simulink model "exp4"  (R2019a)
settings: Solver=ode45  StartTime=0.0  StopTime=10.0  RelTol=1e-3
values from neighbouring files (symbols this model uses):
  Kd = 0.1    [launcher.m]
  Kdp = 0.1    [launcher.m]
  Ki = 0.2    [launcher.m]
  Kip = 0.2    [launcher.m]
  Kp = 5.0    (= 5)    [launcher.m]
  Kpp = 5.0    (= 5)    [launcher.m]
settings Model: Creator=hlf  LastModifiedBy=Aaron
settings DataIOCC: SaveFormat=StructureWithTime
settings OptimizationCC: LifeSpan=inf
settings DebuggingCC: SFExecutionAtInitializationDiag=none  ArithmeticOperatorsInVariantConditions=warning
settings HardwareCC: ProdBitPerSizeT=32  ProdBitPerPtrDiffT=32  ProdWordSize=32  ProdHWDeviceType=Specified
settings CodeAppCC: StateflowObjectComments=on

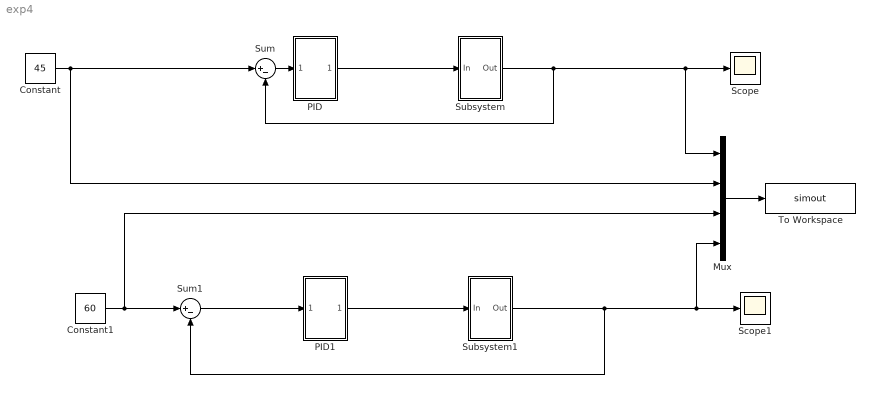
== system exp4 ==
  Constant : Constant  Value=45
  Constant1 : Constant  Value=60
  Mux : Mux
  PID : Subsystem
  PID1 : Subsystem
  Scope : Scope
  Scope1 : Scope
  Subsystem : Subsystem  mask{Ka=0.004, Kf=0.25, Vm=10e-6, Dm=1.75e-5, Kq=0.043, betae=7e8, Kce=3e-13, Jt=0.0167}
  Subsystem1 : Subsystem  mask{Ka=0.004, Kf=0.25, Vm=10e-6, Dm=1.75e-5, Kq=0.043, betae=7e8, Kce=3e-13, Jt=0.0167}
  Sum : Sum  Inputs=|+-
  Sum1 : Sum  Inputs=|+-
  To Workspace : ToWorkspace  VariableName=simout  SaveFormat=Timeseries  SampleTime=-1
  wires:
  Sum/1 -> PID/1(In1)
  PID/1(Out1) -> Subsystem/1(In)
  Subsystem1/1(Out) -> Sum1/2, Mux/4, Scope1/1
  PID1/1(Out1) -> Subsystem1/1(In)
  Sum1/1 -> PID1/1(In1)
  Constant1/1 -> Mux/3, Sum1/1
  Subsystem/1(Out) -> Mux/1, Scope/1, Sum/2
  Mux/1 -> To Workspace/1
  Constant/1 -> Sum/1, Mux/2

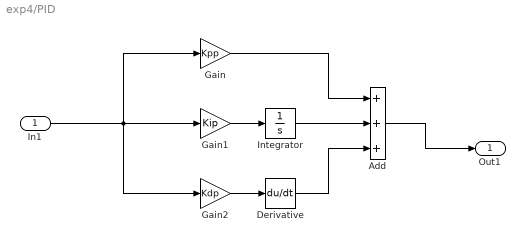
== system exp4/PID ==
  In1 : Inport
  Add : Sum  Inputs=+++
  Derivative : Derivative
  Gain : Gain  Gain=Kpp
  Gain1 : Gain  Gain=Kip
  Gain2 : Gain  Gain=Kdp
  Integrator : Integrator
  Out1 : Outport
  wires:
  Derivative/1 -> Add/3
  In1/1 -> Gain2/1, Gain/1, Gain1/1
  Gain2/1 -> Derivative/1
  Add/1 -> Out1/1
  Gain/1 -> Add/1
  Integrator/1 -> Add/2
  Gain1/1 -> Integrator/1

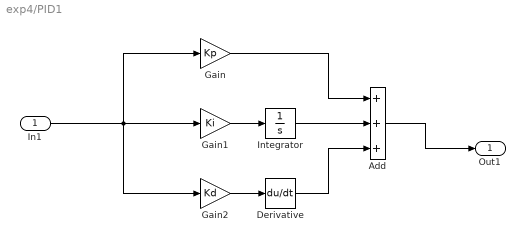
== system exp4/PID1 ==
  In1 : Inport
  Add : Sum  Inputs=+++
  Derivative : Derivative
  Gain : Gain  Gain=Kp
  Gain1 : Gain  Gain=Ki
  Gain2 : Gain  Gain=Kd
  Integrator : Integrator
  Out1 : Outport
  wires:
  Derivative/1 -> Add/3
  In1/1 -> Gain2/1, Gain/1, Gain1/1
  Gain2/1 -> Derivative/1
  Add/1 -> Out1/1
  Gain/1 -> Add/1
  Integrator/1 -> Add/2
  Gain1/1 -> Integrator/1

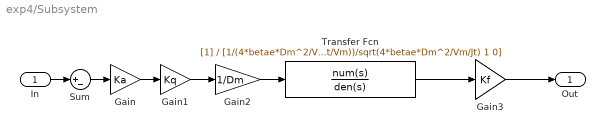
== system exp4/Subsystem ==
  In : Inport
  Gain : Gain  Gain=Ka
  Gain1 : Gain  Gain=Kq
  Gain2 : Gain  Gain=1/Dm
  Gain3 : Gain  Gain=Kf
  Sum : Sum  Inputs=|+-
  Transfer Fcn : TransferFcn  Denominator=[1/(4*betae*Dm^2/Vm/Jt) (2*Kce/Dm*sqrt(betae*Jt/Vm))/sqrt(4*betae*Dm^2/Vm/Jt) 1 0]
  Out : Outport
  wires:
  In/1 -> Sum/1
  Gain1/1 -> Gain2/1
  Gain/1 -> Gain1/1
  Sum/1 -> Gain/1
  Gain2/1 -> Transfer Fcn/1
  Transfer Fcn/1 -> Gain3/1
  Gain3/1 -> Out/1

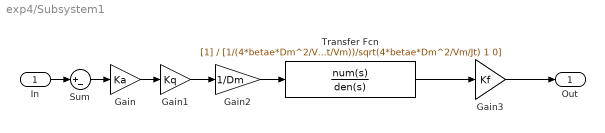
== system exp4/Subsystem1 ==
  In : Inport
  Gain : Gain  Gain=Ka
  Gain1 : Gain  Gain=Kq
  Gain2 : Gain  Gain=1/Dm
  Gain3 : Gain  Gain=Kf
  Sum : Sum  Inputs=|+-
  Transfer Fcn : TransferFcn  Denominator=[1/(4*betae*Dm^2/Vm/Jt) (2*Kce/Dm*sqrt(betae*Jt/Vm))/sqrt(4*betae*Dm^2/Vm/Jt) 1 0]
  Out : Outport
  wires:
  In/1 -> Sum/1
  Gain1/1 -> Gain2/1
  Gain/1 -> Gain1/1
  Sum/1 -> Gain/1
  Gain2/1 -> Transfer Fcn/1
  Transfer Fcn/1 -> Gain3/1
  Gain3/1 -> Out/1
